simulink model "Assignment_1_Group_11_Simulink_model_V1"  (R2018a)
settings: Solver=VariableStepAuto  StartTime=0.0  StopTime=10  RelTol=1e-3
settings Model: Creator=Admin  LastModifiedBy=Admin

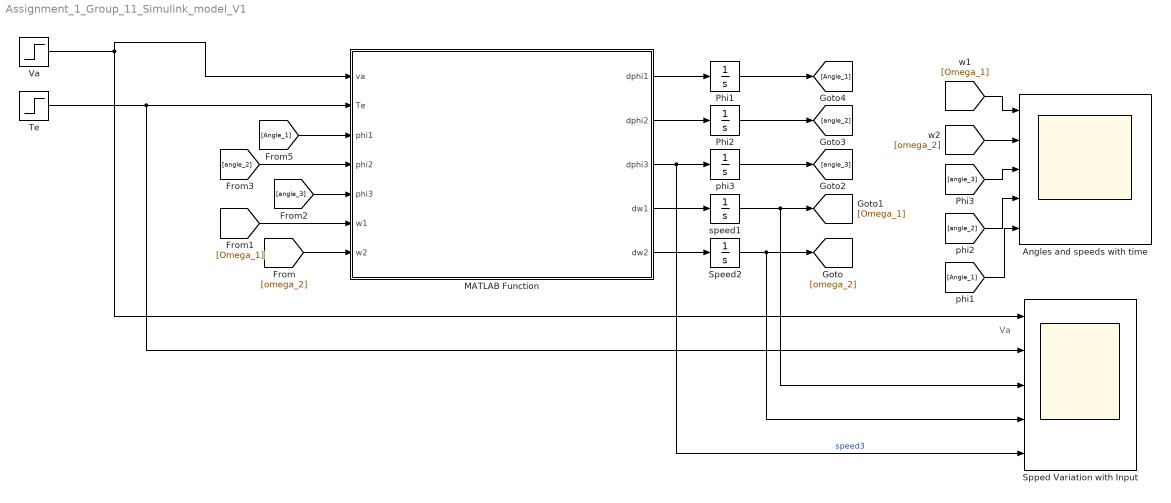
== system Assignment_1_Group_11_Simulink_model_V1 ==
  note: Va
  Angles and speeds with time : Scope  NumInputPorts=5
  MATLAB Function : MATLAB Function  TreatAsAtomicUnit=on
  Phi1 : Integrator
  Phi2 : Integrator
  Speed2 : Integrator
  Spped Variation with Input : Scope  NumInputPorts=5
  "Te " : Step  Time=4  After=-0.1  SampleTime=0
  "Va " : Step  After=10  SampleTime=0
  phi3 : Integrator
  speed1 : Integrator
  wires:
  "Te "/1 -> Spped Variation with Input/2, MATLAB Function/2(Te)
  "Va "/1 -> MATLAB Function/1(va), Spped Variation with Input/1
  MATLAB Function/1(dphi1) -> Phi1/1
  MATLAB Function/2(dphi2) -> Phi2/1
  MATLAB Function/3(dphi3) -> Spped Variation with Input/5, phi3/1  "speed3"
  MATLAB Function/4(dw1) -> speed1/1
  MATLAB Function/5(dw2) -> Speed2/1
  Speed2/1 -> Spped Variation with Input/4, [omega_2]
  [omega_2] -> MATLAB Function/7(w2)
  speed1/1 -> Spped Variation with Input/3, [Omega_1]
  [Omega_1] -> MATLAB Function/6(w1)
  phi3/1 -> [angle_3]
  [angle_3] -> MATLAB Function/5(phi3)
  Phi2/1 -> [angle_2]
  [angle_2] -> MATLAB Function/4(phi2)
  Phi1/1 -> [Angle_1]
  [Angle_1] -> MATLAB Function/3(phi1)
  [angle_2] -> Angles and speeds with time/4
  [angle_3] -> Angles and speeds with time/3
  [omega_2] -> Angles and speeds with time/2
  [Omega_1] -> Angles and speeds with time/1
  [Angle_1] -> Angles and speeds with time/5

== matlab function Assignment_1_Group_11_Simulink_model_V1/MATLAB Function ==
  data: va input; dphi1 output; Te input; phi1 input; phi2 input; phi3 input; w1 input; w2 input; dphi2 output; dphi3 output; dw1 output; dw2 output
function [dphi1,dphi2,dphi3,dw1,dw2] = fcn(va, Te,phi1,phi2,phi3,w1,w2)

R = 1;
ke = 0.1;
kt = ke;
j1 = 10e-5;
j2 = 4*j1;
B = 2*10e-3
D1 = 20;
D2 = 2;


dw1 = ((-kt*ke*w1)/(R*j1))- ((D1/j1)*(phi1 -phi2))+((va*kt)/(j1*R));
dw2 = ((D1/j2)*(phi1 - phi2)) - ((D2/j2)*(phi2-phi3));
dphi1 = w1;
dphi2 = w2;
dphi3 = ((D2/B)*(phi2 - phi3))+ (Te/B)
end
